simulink model "threeexpbi"  (R2017a)
settings: Solver=FixedStepDiscrete  StartTime=0.0  StopTime=Inf  FixedStep=0.01  RelTol=1e-3  EnableMultiTasking=on
settings Model: Creator=eruffaldi  LastModifiedBy=eruffaldi
settings OptimizationCC: LifeSpan=inf
settings DebuggingCC: SFUnexpectedBacktrackingDiag=warning  SFNoUnconditionalDefaultTransitionDiag=warning  SFExecutionAtInitializationDiag=none
settings GRTTargetCC: TargetLangStandard=C89/C90 (ANSI)  GeneratePreprocessorConditionals=Disable all
settings ConfigComp: CovMetricSettings=dw  CovHtmlReporting=on  CovSaveCumulativeToWorkspaceVar=on  CovSaveSingleToWorkspaceVar=on  CovExternalEMLEnable=off

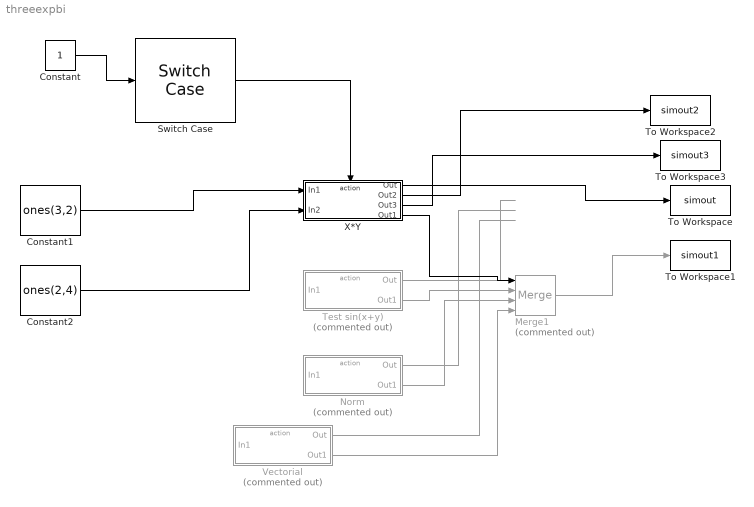
== system threeexpbi ==
  Constant : Constant
  Constant1 : Constant  Value=ones(3,2)
  Constant2 : Constant  Value=ones(2,4)
  Merge1 : Merge  Commented=on  Inputs=4
  Norm : Subsystem  Commented=on  TreatAsAtomicUnit=on
  Switch Case : SwitchCase  ShowDefaultCase=off
  Test sin(x+y) : Subsystem  Commented=on  TreatAsAtomicUnit=on
  To Workspace : ToWorkspace  VariableName=simout  SaveFormat=Timeseries  SampleTime=-1
  To Workspace1 : ToWorkspace  VariableName=simout1  SaveFormat=Timeseries  SampleTime=-1
  To Workspace2 : ToWorkspace  VariableName=simout2  SaveFormat=Timeseries  SampleTime=-1
  To Workspace3 : ToWorkspace  VariableName=simout3  SaveFormat=Timeseries  SampleTime=-1
  Vectorial : Subsystem  Commented=on  TreatAsAtomicUnit=on
  X*Y : Subsystem  TreatAsAtomicUnit=on
  wires:
  Constant/1 -> Switch Case/1
  Switch Case/1 -> X*Y/Action
  X*Y/1(Out) -> To Workspace/1
  Merge1/1 -> To Workspace1/1
  Test sin(x+y)/1(Out) -> ?
  Norm/1(Out) -> ?
  Vectorial/1(Out) -> ?
  X*Y/4(Out1) -> Merge1/1
  Test sin(x+y)/2(Out1) -> Merge1/2
  Norm/2(Out1) -> Merge1/3
  Vectorial/2(Out1) -> Merge1/4
  Constant1/1 -> X*Y/1(In1)
  Constant2/1 -> X*Y/2(In2)
  X*Y/2(Out2) -> To Workspace2/1
  X*Y/3(Out3) -> To Workspace3/1

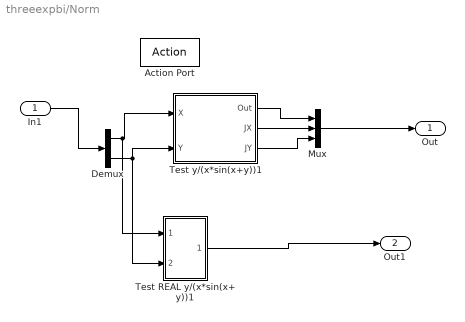
== system threeexpbi/Norm ==
  In1 : Inport
  Action Port : ActionPort
  Demux : Demux  Outputs=2
  Mux : Mux  Inputs=3
  Test REAL y/(x*sin(x+y))1 : Subsystem
  Test y/(x*sin(x+y))1 : Subsystem
  Out : Outport
  Out1 : Outport  Port=2
  wires:
  Demux/2 -> Test y/(x*sin(x+y))1/2(Y), Test REAL y/(x*sin(x+y))1/2(In2)
  In1/1 -> Demux/1
  Demux/1 -> Test y/(x*sin(x+y))1/1(X), Test REAL y/(x*sin(x+y))1/1(In1)
  Test y/(x*sin(x+y))1/1(Out) -> Mux/1
  Test y/(x*sin(x+y))1/2(JX) -> Mux/2
  Test y/(x*sin(x+y))1/3(JY) -> Mux/3
  Mux/1 -> Out/1
  Test REAL y/(x*sin(x+y))1/1(Out1) -> Out1/1

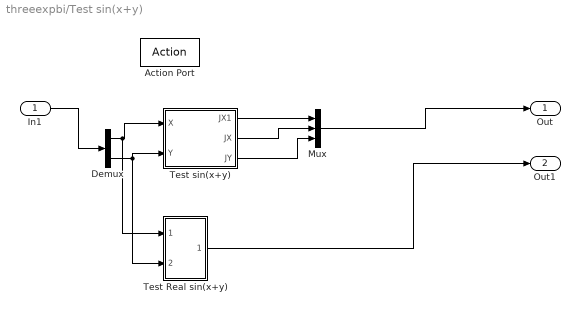
== system threeexpbi/Test sin(x+y) ==
  In1 : Inport
  Action Port : ActionPort
  Demux : Demux  Outputs=2
  Mux : Mux  Inputs=3
  Test Real sin(x+y) : Subsystem
  Test sin(x+y) : Subsystem
  Out : Outport
  Out1 : Outport  Port=2
  wires:
  Demux/2 -> Test Real sin(x+y)/2(In2), Test sin(x+y)/2(Y)
  In1/1 -> Demux/1
  Demux/1 -> Test Real sin(x+y)/1(In1), Test sin(x+y)/1(X)
  Test sin(x+y)/1(JX1) -> Mux/1
  Test sin(x+y)/2(JX) -> Mux/2
  Test sin(x+y)/3(JY) -> Mux/3
  Mux/1 -> Out/1
  Test Real sin(x+y)/1(Out1) -> Out1/1

== system threeexpbi/Vectorial ==
  In1 : Inport
  Action Port : ActionPort
  Demux : Demux  Outputs=2
  Mux : Mux  Inputs=3
  Test REAL y/(x*sin(x+y))1 : Subsystem
  Test y/(x*sin(x+y))1 : Subsystem
  Out : Outport
  Out1 : Outport  Port=2
  wires:
  Demux/2 -> Test y/(x*sin(x+y))1/2(Y), Test REAL y/(x*sin(x+y))1/2(In2)
  In1/1 -> Demux/1
  Demux/1 -> Test y/(x*sin(x+y))1/1(X), Test REAL y/(x*sin(x+y))1/1(In1)
  Test y/(x*sin(x+y))1/1(Out) -> Mux/1
  Test y/(x*sin(x+y))1/2(JX) -> Mux/2
  Test y/(x*sin(x+y))1/3(JY) -> Mux/3
  Mux/1 -> Out/1
  Test REAL y/(x*sin(x+y))1/1(Out1) -> Out1/1

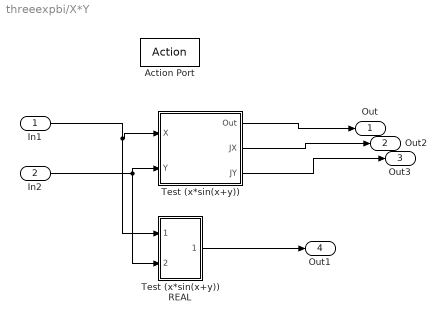
== system threeexpbi/X*Y ==
  In1 : Inport
  In2 : Inport  Port=2
  Action Port : ActionPort  ActionType=case
  Test (x*sin(x+y)) : Subsystem
  Test (x*sin(x+y)) REAL : Subsystem
  Out : Outport
  Out2 : Outport  Port=2
  Out3 : Outport  Port=3
  Out1 : Outport  Port=4
  wires:
  In2/1 -> Test (x*sin(x+y))/2(Y), Test (x*sin(x+y)) REAL/2(In2)
  In1/1 -> Test (x*sin(x+y)) REAL/1(In1), Test (x*sin(x+y))/1(X)
  Test (x*sin(x+y)) REAL/1(Out1) -> Out1/1
  Test (x*sin(x+y))/1(Out) -> Out/1
  Test (x*sin(x+y))/2(JX) -> Out2/1
  Test (x*sin(x+y))/3(JY) -> Out3/1

== system threeexpbi/Norm/Test REAL y//(x*sin(x+y))1 ==
  In1 : Inport
  In2 : Inport  Port=2
  Fcn3 : Fcn  Expr=sqrt(u(1)*u(1)+u(2)*u(2))
  Fcn4 : Fcn  Expr=u(1)/(u(1)^2 + u(2)^2)^(1/2)
  Fcn5 : Fcn  Expr=u(2)/(u(1)^2 + u(2)^2)^(1/2)
  Mux : Mux  Inputs=2
  Mux1 : Mux  Inputs=3
  Out1 : Outport
  wires:
  Fcn5/1 -> Mux1/3
  Fcn4/1 -> Mux1/2
  Fcn3/1 -> Mux1/1
  Mux1/1 -> Out1/1
  In1/1 -> Mux/1
  In2/1 -> Mux/2
  Mux/1 -> Fcn5/1, Fcn4/1, Fcn3/1

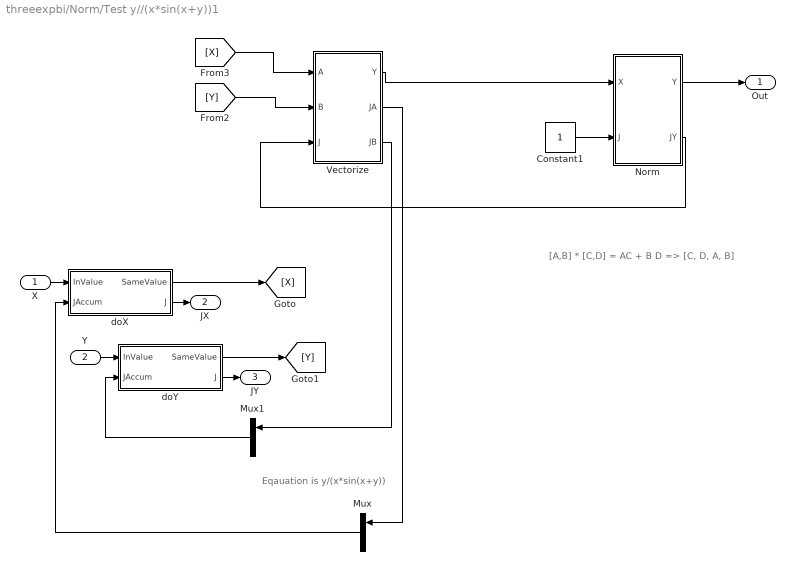
== system threeexpbi/Norm/Test y//(x*sin(x+y))1 ==
  note: [A,B] * [C,D] = AC + B D => [C, D, A, B]
  note: Eqauation is y/(x*sin(x+y))
  X : Inport
  Y : Inport  Port=2
  Constant1 : Constant
  Mux : Mux  Inputs=2
  Mux1 : Mux  Inputs=2
  Norm : Subsystem
  Vectorize : Subsystem
  doX : Subsystem
  doY : Subsystem
  Out : Outport
  JX : Outport  Port=2
  JY : Outport  Port=3
  wires:
  doY/1(SameValue) -> [Y]
  Mux/1 -> doX/2(JAccum)
  Mux1/1 -> doY/2(JAccum)
  Y/1 -> doY/1(InValue)
  doY/2(J) -> JY/1
  doX/1(SameValue) -> [X]
  doX/2(J) -> JX/1
  X/1 -> doX/1(InValue)
  Norm/1(Y) -> Out/1
  [X] -> Vectorize/1(A)
  [Y] -> Vectorize/2(B)
  Vectorize/1(Y) -> Norm/1(X)
  Constant1/1 -> Norm/2(J)
  Norm/2(JY) -> Vectorize/3(J)
  Vectorize/2(JA) -> Mux/1
  Vectorize/3(JB) -> Mux1/1

== system threeexpbi/Test sin(x+y)/Test Real sin(x+y) ==
  In1 : Inport
  In2 : Inport  Port=2
  Fcn : Fcn  Expr=sin(u(1) + u(2))
  Fcn1 : Fcn  Expr=cos(u(1) + u(2))
  Fcn2 : Fcn  Expr=cos(u(1) + u(2))
  Mux1 : Mux  Inputs=3
  Mux2 : Mux  Inputs=2
  Out1 : Outport
  wires:
  Fcn1/1 -> Mux1/2
  Fcn/1 -> Mux1/1
  Mux1/1 -> Out1/1
  Mux2/1 -> Fcn2/1, Fcn1/1, Fcn/1
  Fcn2/1 -> Mux1/3
  In1/1 -> Mux2/1
  In2/1 -> Mux2/2

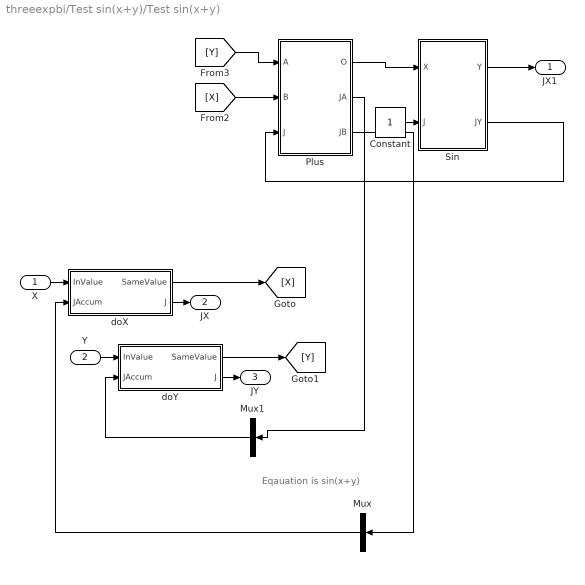
== system threeexpbi/Test sin(x+y)/Test sin(x+y) ==
  note: Eqauation is sin(x+y)
  X : Inport
  Y : Inport  Port=2
  Constant : Constant
  Mux : Mux  Inputs=1
  Mux1 : Mux  Inputs=1
  "Plus " : Subsystem
  Sin : Subsystem
  doX : Subsystem
  doY : Subsystem
  JX1 : Outport
  JX : Outport  Port=2
  JY : Outport  Port=3
  wires:
  [Y] -> "Plus "/1(A)
  doY/1(SameValue) -> [Y]
  Mux/1 -> doX/2(JAccum)
  "Plus "/1(O) -> Sin/1(X)
  Mux1/1 -> doY/2(JAccum)
  Y/1 -> doY/1(InValue)
  "Plus "/3(JB) -> Mux/1
  "Plus "/2(JA) -> Mux1/1
  Sin/2(JY) -> "Plus "/3(J)
  doY/2(J) -> JY/1
  doX/1(SameValue) -> [X]
  doX/2(J) -> JX/1
  X/1 -> doX/1(InValue)
  [X] -> "Plus "/2(B)
  Sin/1(Y) -> JX1/1
  Constant/1 -> Sin/2(J)

== system threeexpbi/Vectorial/Test REAL y//(x*sin(x+y))1 ==
  In1 : Inport
  In2 : Inport  Port=2
  Fcn3 : Fcn  Expr=abs(u(1)+u(2))
  Fcn4 : Fcn  Expr=sign(u(1) + u(2))
  Fcn5 : Fcn  Expr=sign(u(1) + u(2))
  Mux : Mux  Inputs=2
  Mux1 : Mux  Inputs=3
  Out1 : Outport
  wires:
  Fcn5/1 -> Mux1/3
  Fcn4/1 -> Mux1/2
  Fcn3/1 -> Mux1/1
  Mux1/1 -> Out1/1
  In1/1 -> Mux/1
  In2/1 -> Mux/2
  Mux/1 -> Fcn5/1, Fcn4/1, Fcn3/1

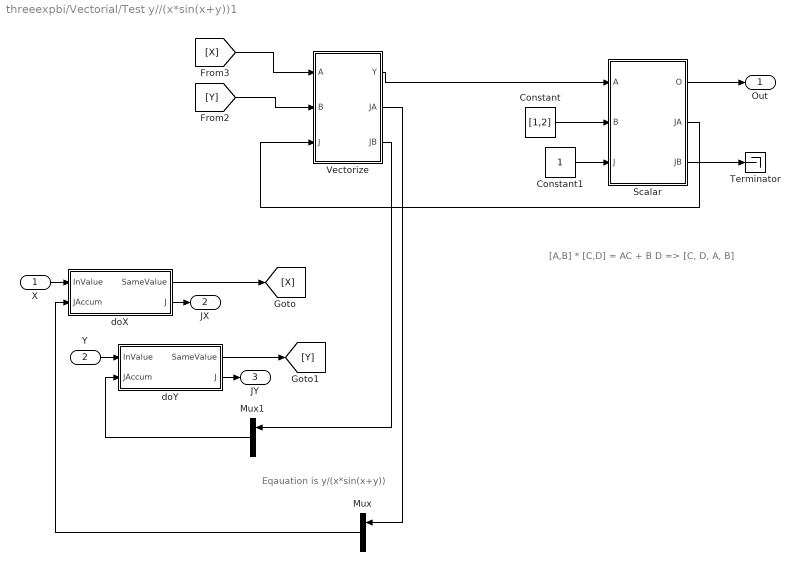
== system threeexpbi/Vectorial/Test y//(x*sin(x+y))1 ==
  note: [A,B] * [C,D] = AC + B D => [C, D, A, B]
  note: Eqauation is y/(x*sin(x+y))
  X : Inport
  Y : Inport  Port=2
  Constant : Constant  Value=[1,2]
  Constant1 : Constant
  Mux : Mux  Inputs=2
  Mux1 : Mux  Inputs=2
  Scalar : Subsystem
  Terminator : Terminator
  Vectorize : Subsystem
  doX : Subsystem
  doY : Subsystem
  Out : Outport
  JX : Outport  Port=2
  JY : Outport  Port=3
  wires:
  doY/1(SameValue) -> [Y]
  Mux/1 -> doX/2(JAccum)
  Mux1/1 -> doY/2(JAccum)
  Y/1 -> doY/1(InValue)
  doY/2(J) -> JY/1
  doX/1(SameValue) -> [X]
  doX/2(J) -> JX/1
  X/1 -> doX/1(InValue)
  Scalar/1(O) -> Out/1
  [X] -> Vectorize/1(A)
  [Y] -> Vectorize/2(B)
  Constant/1 -> Scalar/2(B)
  Vectorize/1(Y) -> Scalar/1(A)
  Scalar/3(JB) -> Terminator/1
  Constant1/1 -> Scalar/3(J)
  Scalar/2(JA) -> Vectorize/3(J)
  Vectorize/2(JA) -> Mux/1
  Vectorize/3(JB) -> Mux1/1

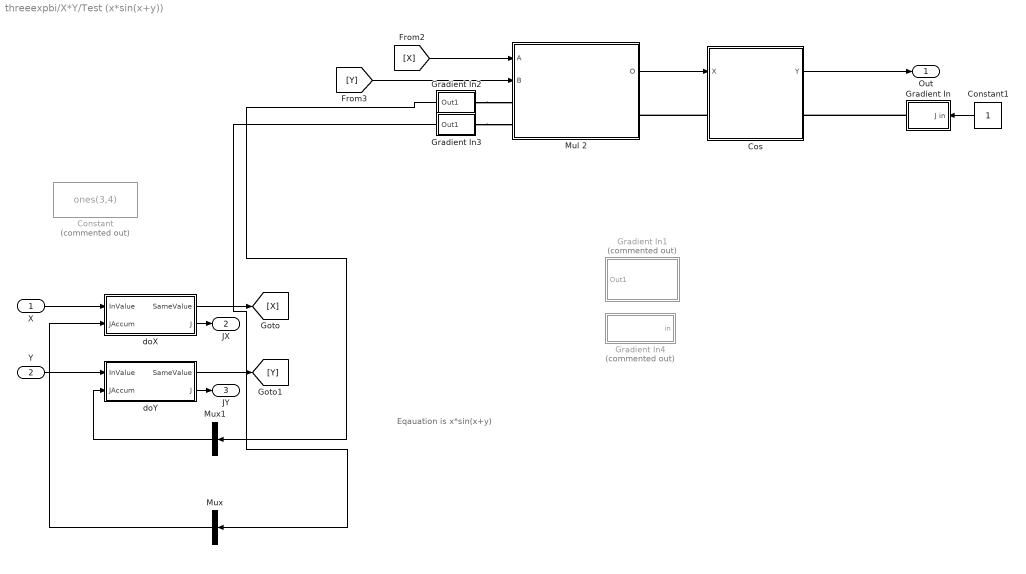
== system threeexpbi/X*Y/Test (x*sin(x+y)) ==
  note: Eqauation is x*sin(x+y)
  X : Inport
  Y : Inport  Port=2
  Constant : Constant  Commented=on  Value=ones(3,4)
  Constant1 : Constant
  Cos : Subsystem
  Gradient In : Subsystem
  Gradient In1 : Subsystem  Commented=on
  Gradient In2 : Subsystem
  Gradient In3 : Subsystem
  Gradient In4 : Subsystem  Commented=on
  Mul 2 : Subsystem
  Mux : Mux  Inputs=1
  Mux1 : Mux  Inputs=1
  doX : Subsystem
  doY : Subsystem
  Out : Outport
  JX : Outport  Port=2
  JY : Outport  Port=3
  wires:
  doY/1(SameValue) -> [Y]
  Mux/1 -> doX/2(JAccum)
  Mux1/1 -> doY/2(JAccum)
  Y/1 -> doY/1(InValue)
  doY/2(J) -> JY/1
  doX/1(SameValue) -> [X]
  doX/2(J) -> JX/1
  X/1 -> doX/1(InValue)
  [X] -> Mul 2/1(A)
  [Y] -> Mul 2/2(B)
  Mul 2/1(O) -> Cos/1(X)
  Cos/1(Y) -> Out/1
  Constant1/1 -> Gradient In/1(J in)
  Gradient In2/1(Out1) -> Mux1/1
  Gradient In3/1(Out1) -> Mux/1
  connections:
  Cos/LConn1 -- Mul 2/RConn1
  Gradient In/RConn1 -- Cos/RConn1
  Gradient In2/LConn1 -- Mul 2/LConn1
  Gradient In3/LConn1 -- Mul 2/LConn2

== system threeexpbi/X*Y/Test (x*sin(x+y)) REAL ==
  In1 : Inport
  In2 : Inport  Port=2
  Mux1 : Mux  Inputs=1
  Product : Product  Multiplication=Matrix(*)
  Out1 : Outport
  wires:
  Product/1 -> Mux1/1
  Mux1/1 -> Out1/1
  In1/1 -> Product/1
  In2/1 -> Product/2

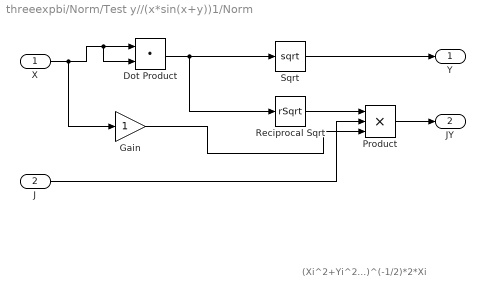
== system threeexpbi/Norm/Test y//(x*sin(x+y))1/Norm ==
  note: (Xi^2+Yi^2...)^(-1/2)*2*Xi
  X : Inport
  J : Inport  Port=2
  Dot Product : DotProduct  InputSameDT=on  OutDataTypeStr=Inherit: Inherit via internal rule
  Gain : Gain
  Product : Product  Inputs=3
  Reciprocal Sqrt : Sqrt  Operator=rSqrt  SaturateOnIntegerOverflow=on
  Sqrt : Sqrt  SaturateOnIntegerOverflow=on
  Y : Outport
  JY : Outport  Port=2
  wires:
  X/1 -> Gain/1, Dot Product/2, Dot Product/1
  J/1 -> Product/2
  Product/1 -> JY/1
  Dot Product/1 -> Reciprocal Sqrt/1, Sqrt/1
  Sqrt/1 -> Y/1
  Reciprocal Sqrt/1 -> Product/1
  Gain/1 -> Product/3

== system threeexpbi/Norm/Test y//(x*sin(x+y))1/Vectorize ==
  A : Inport
  B : Inport  Port=2
  J : Inport  Port=3
  Demux : Demux  Outputs=2
  Mux : Mux  Inputs=2
  Y : Outport
  JA : Outport  Port=2
  JB : Outport  Port=3
  wires:
  Mux/1 -> Y/1
  A/1 -> Mux/1
  B/1 -> Mux/2
  J/1 -> Demux/1
  Demux/1 -> JA/1
  Demux/2 -> JB/1

== system threeexpbi/Norm/Test y//(x*sin(x+y))1/doX ==
  InValue : Inport
  JAccum : Inport  Port=2
  Sum of Elements : Sum  Inputs=+
  SameValue : Outport
  J : Outport  Port=2
  wires:
  InValue/1 -> SameValue/1
  JAccum/1 -> Sum of Elements/1
  Sum of Elements/1 -> J/1

== system threeexpbi/Norm/Test y//(x*sin(x+y))1/doY ==
  InValue : Inport
  JAccum : Inport  Port=2
  Sum of Elements : Sum  Inputs=+
  SameValue : Outport
  J : Outport  Port=2
  wires:
  InValue/1 -> SameValue/1
  JAccum/1 -> Sum of Elements/1
  Sum of Elements/1 -> J/1

== system threeexpbi/Test sin(x+y)/Test sin(x+y)/Plus  ==
  A : Inport
  B : Inport  Port=2
  J : Inport  Port=3
  Add : Sum
  O : Outport
  JA : Outport  Port=2
  JB : Outport  Port=3
  wires:
  Add/1 -> O/1
  A/1 -> Add/1
  B/1 -> Add/2
  J/1 -> JB/1, JA/1

== system threeexpbi/Test sin(x+y)/Test sin(x+y)/Sin ==
  X : Inport
  J : Inport  Port=2
  Product : Product
  Trigonometric Function : Trigonometry
  Trigonometric Function1 : Trigonometry  Operator=cos
  Y : Outport
  JY : Outport  Port=2
  wires:
  Trigonometric Function/1 -> Y/1
  X/1 -> Trigonometric Function1/1, Trigonometric Function/1
  Trigonometric Function1/1 -> Product/1
  J/1 -> Product/2
  Product/1 -> JY/1

== system threeexpbi/Test sin(x+y)/Test sin(x+y)/doX ==
  InValue : Inport
  JAccum : Inport  Port=2
  Sum of Elements : Sum  Inputs=+
  SameValue : Outport
  J : Outport  Port=2
  wires:
  InValue/1 -> SameValue/1
  JAccum/1 -> Sum of Elements/1
  Sum of Elements/1 -> J/1

== system threeexpbi/Test sin(x+y)/Test sin(x+y)/doY ==
  InValue : Inport
  JAccum : Inport  Port=2
  Sum of Elements : Sum  Inputs=+
  SameValue : Outport
  J : Outport  Port=2
  wires:
  InValue/1 -> SameValue/1
  JAccum/1 -> Sum of Elements/1
  Sum of Elements/1 -> J/1

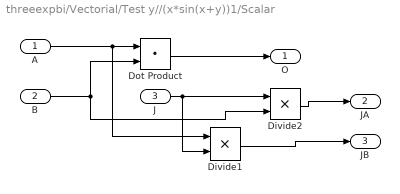
== system threeexpbi/Vectorial/Test y//(x*sin(x+y))1/Scalar ==
  A : Inport
  B : Inport  Port=2
  J : Inport  Port=3
  Divide1 : Product  Inputs=**
  Divide2 : Product  Inputs=**
  Dot Product : DotProduct  InputSameDT=on  OutDataTypeStr=Inherit: Inherit via internal rule
  O : Outport
  JA : Outport  Port=2
  JB : Outport  Port=3
  wires:
  Dot Product/1 -> O/1
  A/1 -> Dot Product/1, Divide1/1
  Divide1/1 -> JB/1
  Divide2/1 -> JA/1
  B/1 -> Dot Product/2, Divide2/2
  J/1 -> Divide1/2, Divide2/1

== system threeexpbi/Vectorial/Test y//(x*sin(x+y))1/Vectorize ==
  A : Inport
  B : Inport  Port=2
  J : Inport  Port=3
  Demux : Demux  Outputs=2
  Mux : Mux  Inputs=2
  Y : Outport
  JA : Outport  Port=2
  JB : Outport  Port=3
  wires:
  Mux/1 -> Y/1
  A/1 -> Mux/1
  B/1 -> Mux/2
  J/1 -> Demux/1
  Demux/1 -> JA/1
  Demux/2 -> JB/1

== system threeexpbi/Vectorial/Test y//(x*sin(x+y))1/doX ==
  InValue : Inport
  JAccum : Inport  Port=2
  Sum of Elements : Sum  Inputs=+
  SameValue : Outport
  J : Outport  Port=2
  wires:
  InValue/1 -> SameValue/1
  JAccum/1 -> Sum of Elements/1
  Sum of Elements/1 -> J/1

== system threeexpbi/Vectorial/Test y//(x*sin(x+y))1/doY ==
  InValue : Inport
  JAccum : Inport  Port=2
  Sum of Elements : Sum  Inputs=+
  SameValue : Outport
  J : Outport  Port=2
  wires:
  InValue/1 -> SameValue/1
  JAccum/1 -> Sum of Elements/1
  Sum of Elements/1 -> J/1

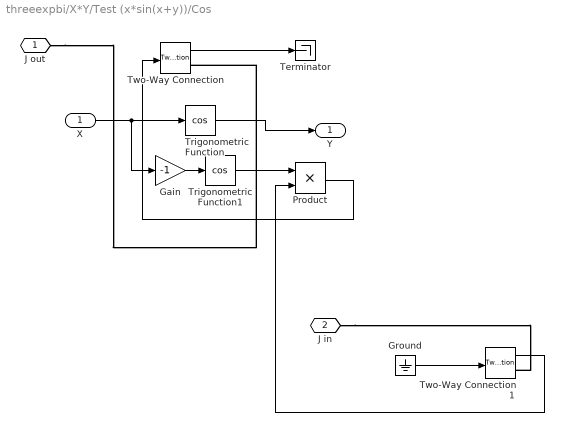
== system threeexpbi/X*Y/Test (x*sin(x+y))/Cos ==
  X : Inport
  Gain : Gain  Gain=-1
  Ground : Ground
  Product : Product
  Terminator : Terminator
  Trigonometric Function : Trigonometry  Operator=cos
  Trigonometric Function1 : Trigonometry  Operator=cos
  Two-Way Connection : TwoWayConnection
  Two-Way Connection1 : TwoWayConnection
  J out : PMIOPort  Port=1  Side=Left
  J in : PMIOPort  Port=2  Side=Right
  Y : Outport
  wires:
  Trigonometric Function/1 -> Y/1
  X/1 -> Gain/1, Trigonometric Function/1
  Trigonometric Function1/1 -> Product/1
  Product/1 -> Two-Way Connection/1
  Gain/1 -> Trigonometric Function1/1
  Two-Way Connection/1 -> Terminator/1
  Two-Way Connection1/1 -> Product/2
  Ground/1 -> Two-Way Connection1/1
  connections:
  J out/RConn1 -- Two-Way Connection/RConn1
  J in/RConn1 -- Two-Way Connection1/RConn1

== system threeexpbi/X*Y/Test (x*sin(x+y))/Gradient In ==
  J in : Inport
  Terminator : Terminator
  Two-Way Connection : TwoWayConnection
  J out : PMIOPort  Port=1  Side=Right
  wires:
  J in/1 -> Two-Way Connection/1
  Two-Way Connection/1 -> Terminator/1
  connections:
  J out/RConn1 -- Two-Way Connection/RConn1

== system threeexpbi/X*Y/Test (x*sin(x+y))/Gradient In1 ==
  Ground : Ground
  Two-Way Connection : TwoWayConnection
  J out : PMIOPort  Port=1  Side=Left
  Out1 : Outport
  wires:
  Two-Way Connection/1 -> Out1/1
  Ground/1 -> Two-Way Connection/1
  connections:
  J out/RConn1 -- Two-Way Connection/RConn1

== system threeexpbi/X*Y/Test (x*sin(x+y))/Gradient In2 ==
  Ground : Ground
  Two-Way Connection : TwoWayConnection
  J out : PMIOPort  Port=1  Side=Left
  Out1 : Outport
  wires:
  Two-Way Connection/1 -> Out1/1
  Ground/1 -> Two-Way Connection/1
  connections:
  J out/RConn1 -- Two-Way Connection/RConn1

== system threeexpbi/X*Y/Test (x*sin(x+y))/Gradient In3 ==
  Ground : Ground
  Two-Way Connection : TwoWayConnection
  J out : PMIOPort  Port=1  Side=Left
  Out1 : Outport
  wires:
  Two-Way Connection/1 -> Out1/1
  Ground/1 -> Two-Way Connection/1
  connections:
  J out/RConn1 -- Two-Way Connection/RConn1

== system threeexpbi/X*Y/Test (x*sin(x+y))/Gradient In4 ==
  " in" : Inport
  Terminator : Terminator
  Two-Way Connection : TwoWayConnection
  J out : PMIOPort  Port=1  Side=Right
  wires:
  " in"/1 -> Two-Way Connection/1
  Two-Way Connection/1 -> Terminator/1
  connections:
  J out/RConn1 -- Two-Way Connection/RConn1

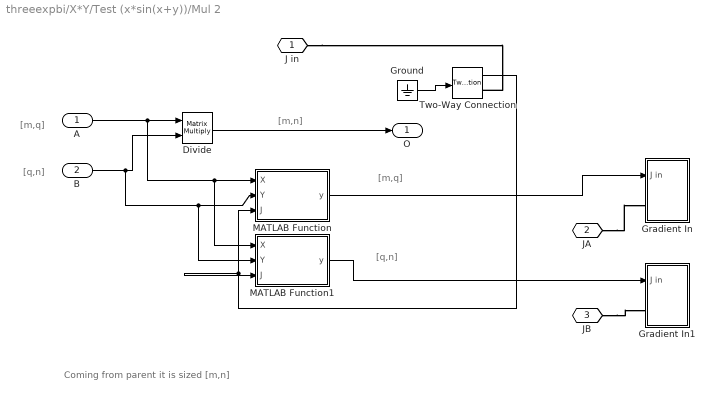
== system threeexpbi/X*Y/Test (x*sin(x+y))/Mul 2 ==
  note: [q,n]
  note: [m,q]
  note: [m,n]
  note: [q,n]
  note: [m,q]
  note: Coming from parent it is sized [m,n]
  A : Inport
  B : Inport  Port=2
  Divide : Product  Inputs=**  Multiplication=Matrix(*)
  Gradient In : Subsystem
  Gradient In1 : Subsystem
  Ground : Ground
  MATLAB Function : MATLAB Function  TreatAsAtomicUnit=on
  MATLAB Function1 : MATLAB Function  TreatAsAtomicUnit=on
  Two-Way Connection : TwoWayConnection
  J in : PMIOPort  Port=1  Side=Right
  JA : PMIOPort  Port=2  Side=Left
  JB : PMIOPort  Port=3  Side=Left
  O : Outport
  wires:
  Divide/1 -> O/1
  A/1 -> MATLAB Function1/1(X), MATLAB Function/1(X), Divide/1
  MATLAB Function1/1(y) -> Gradient In1/1(J in)
  MATLAB Function/1(y) -> Gradient In/1(J in)
  B/1 -> MATLAB Function1/2(Y), MATLAB Function/2(Y), Divide/2
  Two-Way Connection/1 -> MATLAB Function1/3(J), MATLAB Function/3(J)
  Ground/1 -> Two-Way Connection/1
  connections:
  J in/RConn1 -- Two-Way Connection/RConn1
  JA/RConn1 -- Gradient In/LConn1
  JB/RConn1 -- Gradient In1/LConn1

== system threeexpbi/X*Y/Test (x*sin(x+y))/doX ==
  InValue : Inport
  JAccum : Inport  Port=2
  Sum of Elements : Sum  Inputs=+
  SameValue : Outport
  J : Outport  Port=2
  wires:
  InValue/1 -> SameValue/1
  JAccum/1 -> Sum of Elements/1
  Sum of Elements/1 -> J/1

== system threeexpbi/X*Y/Test (x*sin(x+y))/doY ==
  InValue : Inport
  JAccum : Inport  Port=2
  Sum of Elements : Sum  Inputs=+
  SameValue : Outport
  J : Outport  Port=2
  wires:
  InValue/1 -> SameValue/1
  JAccum/1 -> Sum of Elements/1
  Sum of Elements/1 -> J/1

== system threeexpbi/X*Y/Test (x*sin(x+y))/Mul 2/Gradient In ==
  J in : Inport
  Terminator : Terminator
  Two-Way Connection : TwoWayConnection
  J out : PMIOPort  Port=1  Side=Left
  wires:
  J in/1 -> Two-Way Connection/1
  Two-Way Connection/1 -> Terminator/1
  connections:
  J out/RConn1 -- Two-Way Connection/RConn1

== system threeexpbi/X*Y/Test (x*sin(x+y))/Mul 2/Gradient In1 ==
  J in : Inport
  Terminator : Terminator
  Two-Way Connection : TwoWayConnection
  J out : PMIOPort  Port=1  Side=Left
  wires:
  J in/1 -> Two-Way Connection/1
  Two-Way Connection/1 -> Terminator/1
  connections:
  J out/RConn1 -- Two-Way Connection/RConn1

== matlab function threeexpbi/X*Y/Test (x*sin(x+y))/Mul 2/MATLAB Function1 ==
  data: X input; y output; Y input; J input
function y = fcn(X,Y,J)
%#codegen

y = repmat(reshape(sum(X,1),size(X,2),1),1,size(Y,2));
if length(J) == 1
    y = J*y;
else
    y = repmat(sum(J,1),size(Y,1),1).*y;
end

== matlab function threeexpbi/X*Y/Test (x*sin(x+y))/Mul 2/MATLAB Function ==
  data: X input; y output; Y input; J input
function y = fcn(X,Y,J)
%#codegen

y = repmat(reshape(sum(Y,2),1,size(Y,1)),size(X,1),1);
if length(J) == 1
    y = J*y;
else
    y = repmat(sum(J,2),1,size(X,2)).*y;
end
